simulink model "cascade_sim"  (R2015a)
settings: Solver=ode45  StartTime=0.0  StopTime=25  RelTol=1e-3
values from neighbouring files (symbols this model uses):
  s = tf('s')    [ekstranul.m]
libraries: cstblocks x6, simulink x1
settings Model: Creator=morten  LastModifiedBy=roevhat

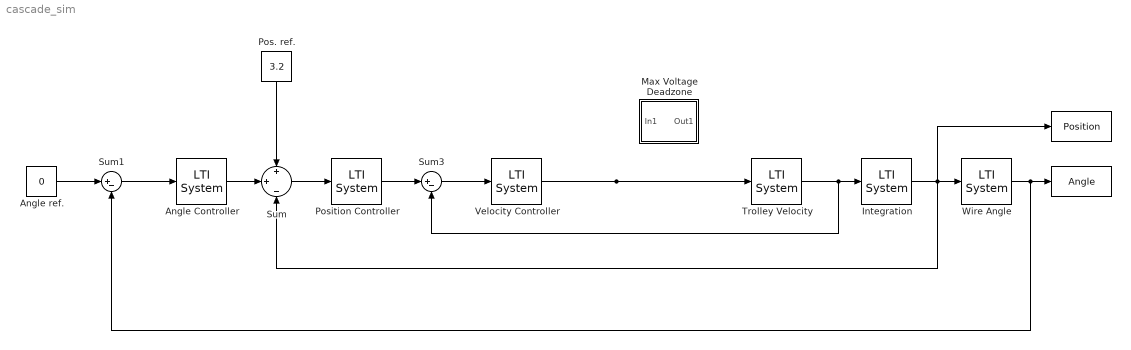
== system cascade_sim ==
  "  " : ToWorkspace  VariableName=Angle  SaveFormat=Timeseries  SampleTime=-1
  "   " : ToWorkspace  VariableName=Position  SaveFormat=Timeseries  SampleTime=-1
  Angle Controller : cstblocks/LTI System  sys=dCa  IC=[]
  Angle ref. : Constant  Value=0
  Integration : cstblocks/LTI System  sys=1/s  IC=[]
  Max Voltage Deadzone : Subsystem
  Pos. ref. : Constant  Value=3.2
  Position Controller : cstblocks/LTI System  sys=Cx  IC=[]
  Sum : Sum  Inputs=+|+|-
  Sum1 : Sum  Inputs=|+-
  Sum3 : Sum  Inputs=|+-
  Trolley Velocity : cstblocks/LTI System  sys=Gx  IC=[]
  Velocity Controller : cstblocks/LTI System  sys=Cv  IC=[]
  Wire Angle : cstblocks/LTI System  sys=W  IC=[]
  wires:
  Velocity Controller/1 -> Trolley Velocity/1
  Integration/1 -> Sum/3, Wire Angle/1, "   "/1
  Trolley Velocity/1 -> Integration/1, Sum3/2
  Wire Angle/1 -> Sum1/2, "  "/1
  Sum/1 -> Position Controller/1
  Sum3/1 -> Velocity Controller/1
  Position Controller/1 -> Sum3/1
  Sum1/1 -> Angle Controller/1
  Angle ref./1 -> Sum1/1
  Angle Controller/1 -> Sum/2
  Pos. ref./1 -> Sum/1

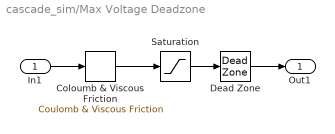
== system cascade_sim/Max Voltage Deadzone ==
  In1 : Inport
  Coloumb & Viscous Friction : simulink/Discontinuities/Coulomb & Viscous Friction  offset=[4.2]  gain=1
  Dead Zone : DeadZone  LowerValue=-4.1  UpperValue=4.1  SaturateOnIntegerOverflow=on
  Saturation : Saturate  UpperLimit=12.5  LowerLimit=-12.5
  Out1 : Outport
  wires:
  Dead Zone/1 -> Out1/1
  Saturation/1 -> Dead Zone/1
  In1/1 -> Coloumb & Viscous Friction/1
  Coloumb & Viscous Friction/1 -> Saturation/1
